simulink model "hematology"  (R2024b)
settings: Solver=VariableStepAuto  StartTime=0.0  StopTime=10.0  RelTol=1e-3
libraries: visionstatistics x1
settings Model: Creator=Hp  LastModifiedBy=Hp

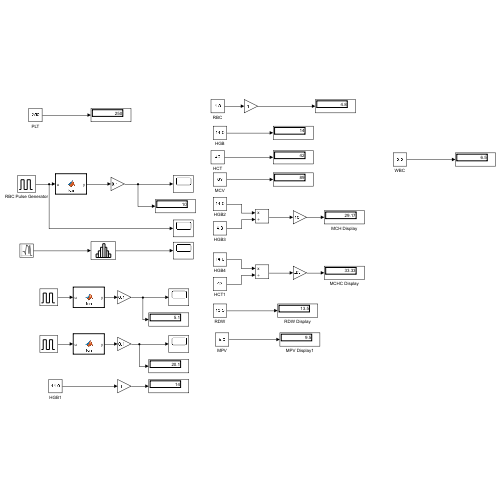
[thumbnail: Simulink's stored preview of the top-level diagram]
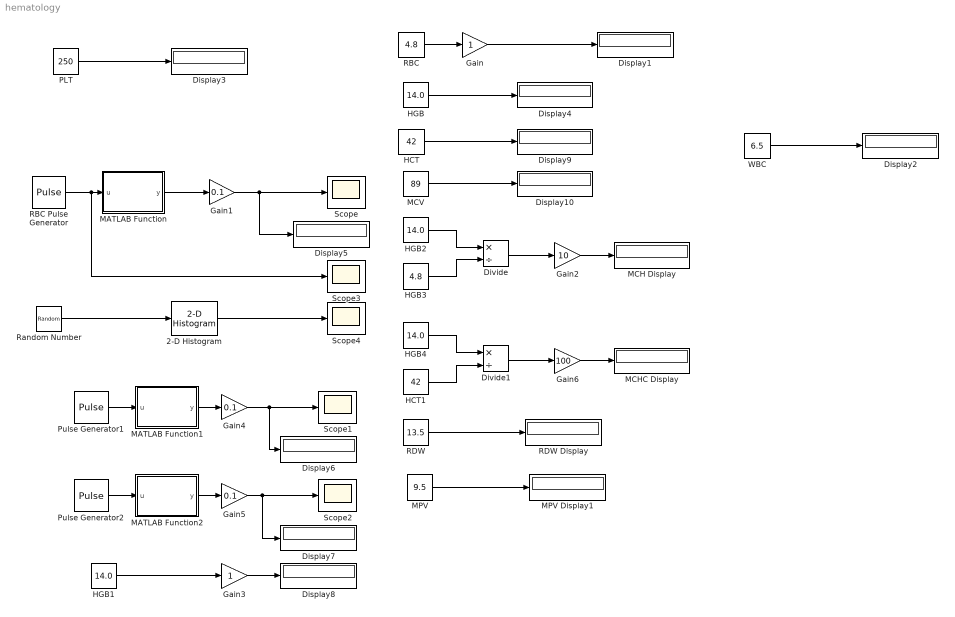
== system hematology ==
  2-D Histogram : visionstatistics/2-D Histogram  umin=0  umax=1  nbins=256  operateOver=Entire input  normalized=off  run=off  reset=on  trigtype=None  Dimension=1  colComp=on  roundingMode=Floor  overflowMode=off
  Display{1..10} (10 alike) : Display
  Divide : Product  Inputs=*/
  Divide1 : Product  Inputs=*/
  Gain : Gain
  Gain1 : Gain  Gain=0.1
  Gain2 : Gain  Gain=10
  Gain3 : Gain
  Gain4 : Gain  Gain=0.1
  Gain5 : Gain  Gain=0.1
  Gain6 : Gain  Gain=100
  HCT : Constant  Value=42
  HCT1 : Constant  Value=42
  HGB{,1..2,4} (4 alike) : Constant  Value=14.0
  HGB3 : Constant  Value=4.8
  MATLAB Function : MATLAB Function  TreatAsAtomicUnit=on
  MATLAB Function1 : MATLAB Function  TreatAsAtomicUnit=on
  MATLAB Function2 : MATLAB Function  TreatAsAtomicUnit=on
  MCH Display : Display
  MCHC Display : Display
  MCV : Constant  Value=89
  MPV : Constant  Value=9.5
  MPV Display1 : Display
  PLT : Constant  Value=250
  Pulse Generator1 : DiscretePulseGenerator  PulseType=Time based  Period=0.2  PulseWidth=10
  Pulse Generator2 : DiscretePulseGenerator  PulseType=Time based  Period=0.05  PulseWidth=10
  RBC : Constant  Value=4.8
  RBC Pulse Generator : DiscretePulseGenerator  PulseType=Time based  Period=0.1  PulseWidth=10  PhaseDelay=0.01
  RDW : Constant  Value=13.5
  RDW Display : Display
  Random Number : RandomNumber  SampleTime=0.1
  Scope{,1..4} (5 alike) : Scope
  WBC : Constant  Value=6.5
  wires:
  RBC/1 -> Gain/1
  WBC/1 -> Display2/1
  PLT/1 -> Display3/1
  HGB/1 -> Display4/1
  Gain/1 -> Display1/1
  RBC Pulse Generator/1 -> Scope3/1, MATLAB Function/1(u)
  MATLAB Function/1(y) -> Gain1/1
  Gain1/1 -> Display5/1, Scope/1
  Pulse Generator1/1 -> MATLAB Function1/1(u)
  MATLAB Function1/1(y) -> Gain4/1
  MATLAB Function2/1(y) -> Gain5/1
  Pulse Generator2/1 -> MATLAB Function2/1(u)
  Gain5/1 -> Display7/1, Scope2/1
  HGB1/1 -> Gain3/1
  Gain3/1 -> Display8/1
  HCT/1 -> Display9/1
  MCV/1 -> Display10/1
  Divide/1 -> Gain2/1
  Gain2/1 -> MCH Display/1
  HGB3/1 -> Divide/2
  HGB2/1 -> Divide/1
  HGB4/1 -> Divide1/1
  HCT1/1 -> Divide1/2
  Divide1/1 -> Gain6/1
  Gain6/1 -> MCHC Display/1
  RDW/1 -> RDW Display/1
  MPV/1 -> MPV Display1/1
  Gain4/1 -> Display6/1, Scope1/1
  Random Number/1 -> 2-D Histogram/1
  2-D Histogram/1 -> Scope4/1

== matlab function hematology/MATLAB Function ==
  data: u input; y output
function y = fcn(u)
persistent count previous

if isempty(count)
    count = 0;
    previous = 0;
end

if u > 0 && previous == 0
    count = count +1;
end

previous = u;
y = count;

== matlab function hematology/MATLAB Function2 ==
  data: u input; y output
function y = fcn(u)
persistent count previous

if isempty(count)
    count = 0;
    previous = 0;
end

if u > 0 && previous == 0
    count = count +1;
end

previous = u;
y = count;

== matlab function hematology/MATLAB Function1 ==
  data: u input; y output
function y = fcn(u)
persistent count previous

if isempty(count)
    count = 0;
    previous = 0;
end

if u > 0 && previous == 0
    count = count +1;
end

previous = u;
y = count;
